simulink model "ex_han2"  (Simulink 8.3)
settings: Solver=ode5  StartTime=0.0  StopTime=409  FixedStep=T  RelTol=1e-3
PreLoadFcn:
  | r=10; h=0.01; T=0.01; bet=[100,65,80]; bet1=[100,10]; aa=[0.75,1.25]; d=0; b=1;
settings Model: Creator=Administrator  LastModifiedBy=Administrator  CovSFcnEnable=on
settings DataIOCC: LimitDataPoints=off
settings OptimizationCC: BooleanDataType=off
settings DebuggingCC: SaveWithParameterizedLinksMsg=none  SignalResolutionControl=TryResolveAllWithWarning  SolverPrmCheckMsg=none  MultiTaskDSMMsg=warning  MultiTaskCondExecSysMsg=none  FrameProcessingCompatibilityMsg=error  StateNameClashWarn=none
settings HardwareCC: TargetUnknown=on

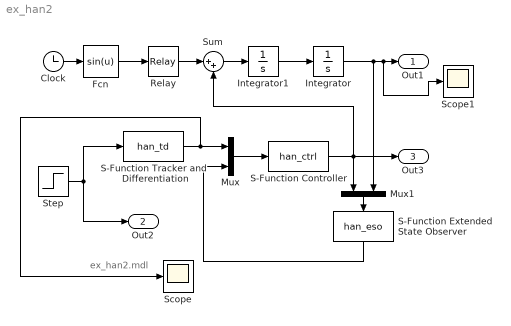
== system ex_han2 ==
  note: ex_han2.mdl
  Clock : Clock
  Fcn : Fcn  Expr=sin(u)
  Integrator : Integrator
  Integrator1 : Integrator
  Mux : Mux  Inputs=2
  Mux1 : Mux  Inputs=2
  Relay : Relay
  S-Function Controller : S-Function  FunctionName=han_ctrl  Parameters=aa,bet1,b,d  EnableBusSupport=off
  S-Function Extended State Observer : S-Function  FunctionName=han_eso  Parameters=d,bet,b,T  EnableBusSupport=off
  S-Function Tracker and  Differentiation : S-Function  FunctionName=han_td  Parameters=r,h,T  EnableBusSupport=off
  Scope : Scope
  Scope1 : Scope
      settings: YMin=9.9965  YMax=10.003
  Step : Step  After=10  SampleTime=0
  Sum : Sum  Inputs=|++  SaturateOnIntegerOverflow=on  InputSameDT=on  OutDataTypeStr=Inherit: Same as first input
  Out1 : Outport
  Out2 : Outport  Port=2
  Out3 : Outport  Port=3
  wires:
  Clock/1 -> Fcn/1
  Sum/1 -> Integrator1/1
  Integrator1/1 -> Integrator/1
  Integrator/1 -> Scope1/1, Out1/1, Mux1/2
  Step/1 -> S-Function Tracker and  Differentiation/1, Out2/1
  S-Function Controller/1 -> Sum/2, Out3/1, Mux1/1
  S-Function Tracker and  Differentiation/1 -> Scope/1, Mux/1
  Mux/1 -> S-Function Controller/1
  S-Function Extended State Observer/1 -> Mux/2
  Fcn/1 -> Relay/1
  Relay/1 -> Sum/1
  Mux1/1 -> S-Function Extended State Observer/1
